simulink model "HA_sys7"  (R2017a)
settings: Solver=FixedStepDiscrete  StartTime=0.0  StopTime=stopTime  RelTol=1e-3
InitFcn:
  | HA_sys7_init
StopFcn:
  | %figure(1)
  | 
  | %subplot(2,1,1)
  | %plot(HA_left_data_out)
  | %title('Left Channel Output')
  | 
  | %subplot(2,1,2)
  | %plot(HA_right_data_out)
  | %title('Right Channel Output')
values from neighbouring files (symbols this model uses):
  Fs = 48000    [HA_sys7_init.m]
  Gain_B1_left = 1    [HA_sys7_init.m]
  Gain_B1_right = 1    [HA_sys7_init.m]
  Gain_B2_left = 1    [HA_sys7_init.m]
  Gain_B2_right = 1    [HA_sys7_init.m]
  Gain_B3_left = 1    [HA_sys7_init.m]
  Gain_B3_right = 1    [HA_sys7_init.m]
  Gain_B4_left = 1    [HA_sys7_init.m]
  Gain_B4_right = 1    [HA_sys7_init.m]
  Gain_B5_left = 1    [HA_sys7_init.m]
  Gain_B5_right = 1    [HA_sys7_init.m]
undefined symbols (not defined in the file or in its folder): FIRBandPass1, FIRBandPass2, FIRBandPass3, FIRBandPass4, FIRBandPass5, FIRDecimator1, FIRDecimator2, FIRDecimator3, FIRDecimator4, FIRDecimator5, FIRInterpolator1, FIRInterpolator2, FIRInterpolator3, FIRInterpolator4, FIRInterpolator5
libraries: dspmlti4 x20, dspsrcs4 x1
settings Model: DataTypeOverride=Off  Creator=The MathWorks, Inc.  LastModifiedBy=Ross_admin
settings DataIOCC: LimitDataPoints=on  SaveFormat=Array  SaveOutput=off  SaveTime=off
settings OptimizationCC: BlockReduction=off  ConditionallyExecuteInputs=off  DefaultParameterBehavior=Inlined  LifeSpan=inf
settings DebuggingCC: AlgebraicLoopMsg=error  SingleTaskRateTransMsg=error  AllowSymbolicDim=off  StrictBusMsg=ErrorOnBusTreatedAsVector  SFUnexpectedBacktrackingDiag=warning  SFNoUnconditionalDefaultTransitionDiag=warning  SFExecutionAtInitializationDiag=none
settings HardwareCC: ProdBitPerPointer=32  ProdBitPerSizeT=32  ProdBitPerPtrDiffT=32  ProdLargestAtomicFloat=None  ProdIntDivRoundTo=Undefined  ProdEndianess=Unspecified  ProdWordSize=32  ProdHWDeviceType=ASIC/FPGA->ASIC/FPGA  ProdEqTarget=off
settings ModelReferenceCC: PropagateSignalLabelsOutOfModel=off
settings GRTTargetCC: TargetLangStandard=C89/C90 (ANSI)  GeneratePreprocessorConditionals=Disable all
settings ConfigComp: CovMetricSettings=dw  CovHtmlReporting=on  CovSaveCumulativeToWorkspaceVar=on  CovSaveSingleToWorkspaceVar=on  CovShowResultsExplorer=off  CovExternalEMLEnable=off

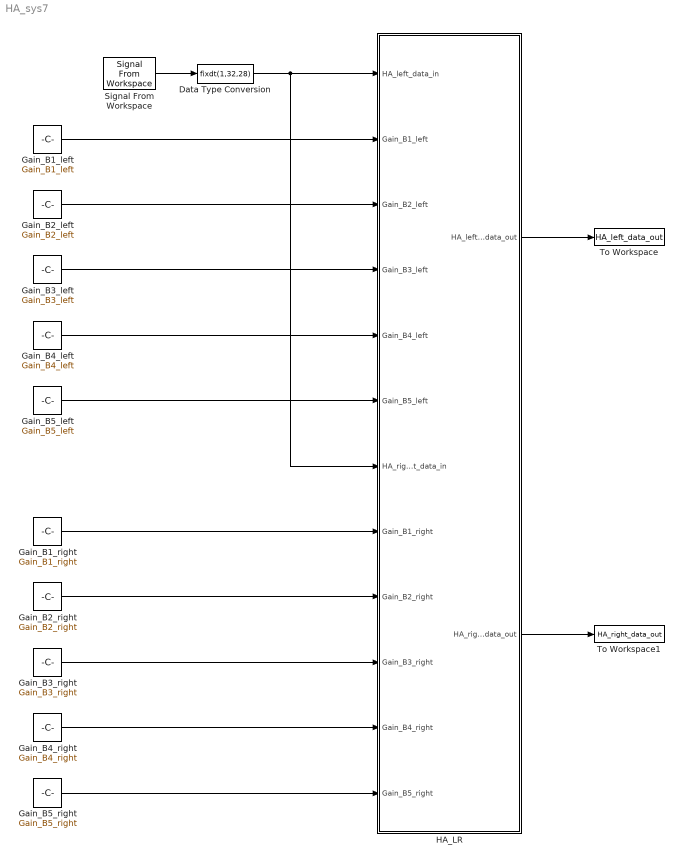
== system HA_sys7 ==
  Data Type Conversion : DataTypeConversion  OutDataTypeStr=fixdt(1,32,28)
  Gain_B1_left : Constant  Value=Gain_B1_left  OutDataTypeStr=fixdt(1,32,16)  SampleTime=-1  LockScale=on
  Gain_B1_right : Constant  Value=Gain_B1_right  OutDataTypeStr=fixdt(1,32,16)  SampleTime=-1  LockScale=on
  Gain_B2_left : Constant  Value=Gain_B2_left  OutDataTypeStr=fixdt(1,32,16)  SampleTime=-1  LockScale=on
  Gain_B2_right : Constant  Value=Gain_B2_right  OutDataTypeStr=fixdt(1,32,16)  SampleTime=-1  LockScale=on
  Gain_B3_left : Constant  Value=Gain_B3_left  OutDataTypeStr=fixdt(1,32,16)  SampleTime=-1  LockScale=on
  Gain_B3_right : Constant  Value=Gain_B3_right  OutDataTypeStr=fixdt(1,32,16)  SampleTime=-1  LockScale=on
  Gain_B4_left : Constant  Value=Gain_B4_left  OutDataTypeStr=fixdt(1,32,16)  SampleTime=-1  LockScale=on
  Gain_B4_right : Constant  Value=Gain_B4_right  OutDataTypeStr=fixdt(1,32,16)  SampleTime=-1  LockScale=on
  Gain_B5_left : Constant  Value=Gain_B5_left  OutDataTypeStr=fixdt(1,32,16)  SampleTime=-1  LockScale=on
  Gain_B5_right : Constant  Value=Gain_B5_right  OutDataTypeStr=fixdt(1,32,16)  SampleTime=-1  LockScale=on
  HA_LR : Subsystem
  Signal From Workspace : dspsrcs4/Signal From Workspace  X=signal_in  Ts=1/Fs  nsamps=1  OutputAfterFinalValue=Setting to zero  ignoreOrWarnInputAndFrameLengths=off  OutputFrames=off
  To Workspace : ToWorkspace  VariableName=HA_left_data_out  SampleTime=-1
      settings: Save2DSignal=2-D array (concatenate along first dimension)
  To Workspace1 : ToWorkspace  VariableName=HA_right_data_out  SampleTime=-1
      settings: Save2DSignal=2-D array (concatenate along first dimension)
  wires:
  Signal From Workspace/1 -> Data Type Conversion/1
  Data Type Conversion/1 -> HA_LR/7(HA_right_data_in), HA_LR/1(HA_left_data_in)
  Gain_B2_left/1 -> HA_LR/3(Gain_B2_left)
  Gain_B3_left/1 -> HA_LR/4(Gain_B3_left)
  Gain_B4_left/1 -> HA_LR/5(Gain_B4_left)
  Gain_B5_left/1 -> HA_LR/6(Gain_B5_left)
  HA_LR/1(HA_left_data_out) -> To Workspace/1
  HA_LR/2(HA_right_data_out) -> To Workspace1/1
  Gain_B1_left/1 -> HA_LR/2(Gain_B1_left)
  Gain_B1_right/1 -> HA_LR/8(Gain_B1_right)
  Gain_B2_right/1 -> HA_LR/9(Gain_B2_right)
  Gain_B4_right/1 -> HA_LR/11(Gain_B4_right)
  Gain_B5_right/1 -> HA_LR/12(Gain_B5_right)
  Gain_B3_right/1 -> HA_LR/10(Gain_B3_right)

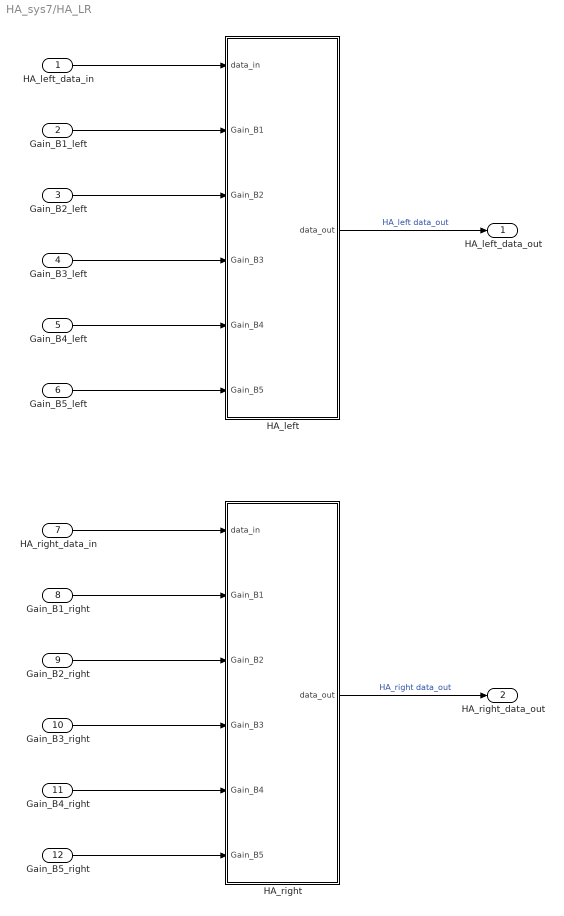
== system HA_sys7/HA_LR ==
  HA_left_data_in : Inport
  Gain_B1_left : Inport  Port=2
  Gain_B2_left : Inport  Port=3
  Gain_B3_left : Inport  Port=4
  Gain_B4_left : Inport  Port=5
  Gain_B5_left : Inport  Port=6
  HA_right_data_in : Inport  Port=7
  Gain_B1_right : Inport  Port=8
  Gain_B2_right : Inport  Port=9
  Gain_B3_right : Inport  Port=10
  Gain_B4_right : Inport  Port=11
  Gain_B5_right : Inport  Port=12
  HA_left : Subsystem
  HA_right : Subsystem
  HA_left_data_out : Outport
  HA_right_data_out : Outport  Port=2
  wires:
  Gain_B5_left/1 -> HA_left/6(Gain_B5)
  Gain_B4_left/1 -> HA_left/5(Gain_B4)
  Gain_B2_left/1 -> HA_left/3(Gain_B2)
  Gain_B3_left/1 -> HA_left/4(Gain_B3)
  Gain_B3_right/1 -> HA_right/4(Gain_B3)
  HA_right_data_in/1 -> HA_right/1(data_in)
  HA_right/1(data_out) -> HA_right_data_out/1  "HA_right data_out"
  Gain_B1_right/1 -> HA_right/2(Gain_B1)
  Gain_B2_right/1 -> HA_right/3(Gain_B2)
  Gain_B4_right/1 -> HA_right/5(Gain_B4)
  Gain_B5_right/1 -> HA_right/6(Gain_B5)
  HA_left_data_in/1 -> HA_left/1(data_in)
  HA_left/1(data_out) -> HA_left_data_out/1  "HA_left data_out"
  Gain_B1_left/1 -> HA_left/2(Gain_B1)

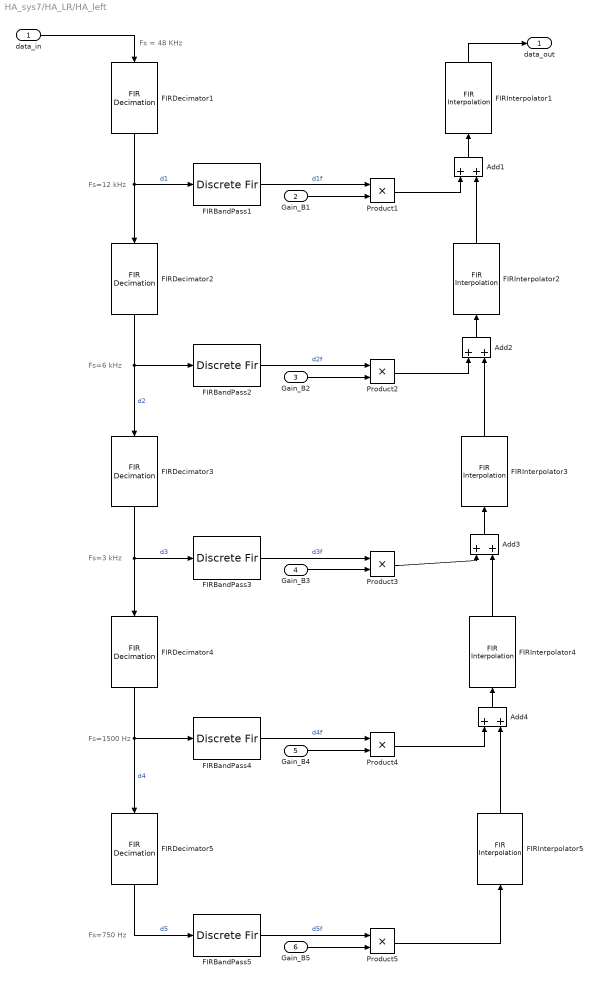
== system HA_sys7/HA_LR/HA_left ==
  note: Fs = 48 KHz
  note: Fs=12 kHz
  note: Fs=6 kHz
  note: Fs=3 kHz
  note: Fs=1500 Hz
  note: Fs=750 Hz
  data_in : Inport
  Gain_B1 : Inport  Port=2  OutDataTypeStr=fixdt(1,32,16)  LockScale=on
  Gain_B2 : Inport  Port=3  OutDataTypeStr=fixdt(1,32,16)  LockScale=on
  Gain_B3 : Inport  Port=4  OutDataTypeStr=fixdt(1,32,16)  LockScale=on
  Gain_B4 : Inport  Port=5  OutDataTypeStr=fixdt(1,32,16)  LockScale=on
  Gain_B5 : Inport  Port=6  OutDataTypeStr=fixdt(1,32,16)  LockScale=on
  Add{1..4} (4 alike) : Sum  SaturateOnIntegerOverflow=on
  FIRBandPass1 : DiscreteFir  Coefficients=FIRBandPass1.FIR_coefficients  AccumDataTypeStr=Inherit: Same as product output  SaturateOnIntegerOverflow=on
  FIRBandPass2 : DiscreteFir  Coefficients=FIRBandPass2.FIR_coefficients  AccumDataTypeStr=Inherit: Same as product output  OutDataTypeStr=FIRBandPass2.numeric_type  SaturateOnIntegerOverflow=on
  FIRBandPass3 : DiscreteFir  Coefficients=FIRBandPass3.FIR_coefficients  AccumDataTypeStr=Inherit: Same as product output  OutDataTypeStr=FIRBandPass2.numeric_type  SaturateOnIntegerOverflow=on
  FIRBandPass4 : DiscreteFir  Coefficients=FIRBandPass4.FIR_coefficients  AccumDataTypeStr=Inherit: Same as product output  OutDataTypeStr=FIRBandPass2.numeric_type  SaturateOnIntegerOverflow=on
  FIRBandPass5 : DiscreteFir  Coefficients=FIRBandPass5.FIR_coefficients  AccumDataTypeStr=Inherit: Same as product output  OutDataTypeStr=FIRBandPass2.numeric_type  SaturateOnIntegerOverflow=on
  FIRDecimator1 : dspmlti4/FIR Decimation  FilterSource=Dialog parameters  h=FIRDecimator1.FIR_coefficients  D=FIRDecimator1.decimation_factor  filtStruct=Direct form  FilterObject=FDECIM  framing=Allow multirate processing  inputOffset=0  outputBufInitCond=0  roundingMode=Floor  overflowMode=on  firstCoeffDataTypeStr=Inherit: Same word length as input  firstCoeffMin=[]  firstCoeffMax=[]  firstCoeffLastDataTypeStr=Inherit: Same word length as input  outputMode=Binary point scaling  outputWordLength=32  outputFracLength=28  outputDataTypeStr=fixdt(1,32,28)  outputMin=[]  outputMax=[]  outputLastDataTypeStr=fixdt(1,32,28)
  FIRDecimator2 : dspmlti4/FIR Decimation  FilterSource=Dialog parameters  h=FIRDecimator2.FIR_coefficients  D=FIRDecimator2.decimation_factor  filtStruct=Direct form  FilterObject=FDECIM  framing=Allow multirate processing  inputOffset=0  outputBufInitCond=0  roundingMode=Floor  overflowMode=on  firstCoeffDataTypeStr=Inherit: Same word length as input  firstCoeffMin=[]  firstCoeffMax=[]  firstCoeffLastDataTypeStr=Inherit: Same word length as input  outputMode=Binary point scaling  outputWordLength=32  outputFracLength=28  outputDataTypeStr=fixdt(1,32,28)  outputMin=[]  outputMax=[]  outputLastDataTypeStr=fixdt(1,32,28)
  FIRDecimator3 : dspmlti4/FIR Decimation  FilterSource=Dialog parameters  h=FIRDecimator3.FIR_coefficients  D=FIRDecimator3.decimation_factor  filtStruct=Direct form  FilterObject=FDECIM  framing=Allow multirate processing  inputOffset=0  outputBufInitCond=0  roundingMode=Floor  overflowMode=on  firstCoeffDataTypeStr=Inherit: Same word length as input  firstCoeffMin=[]  firstCoeffMax=[]  firstCoeffLastDataTypeStr=Inherit: Same word length as input  outputMode=Binary point scaling  outputWordLength=32  outputFracLength=28  outputDataTypeStr=fixdt(1,32,28)  outputMin=[]  outputMax=[]  outputLastDataTypeStr=fixdt(1,32,28)
  FIRDecimator4 : dspmlti4/FIR Decimation  FilterSource=Dialog parameters  h=FIRDecimator4.FIR_coefficients  D=FIRDecimator4.decimation_factor  filtStruct=Direct form  FilterObject=FDECIM  framing=Allow multirate processing  inputOffset=0  outputBufInitCond=0  roundingMode=Floor  overflowMode=on  firstCoeffDataTypeStr=Inherit: Same word length as input  firstCoeffMin=[]  firstCoeffMax=[]  firstCoeffLastDataTypeStr=Inherit: Same word length as input  outputMode=Binary point scaling  outputWordLength=32  outputFracLength=28  outputDataTypeStr=fixdt(1,32,28)  outputMin=[]  outputMax=[]  outputLastDataTypeStr=fixdt(1,32,28)
  FIRDecimator5 : dspmlti4/FIR Decimation  FilterSource=Dialog parameters  h=FIRDecimator5.FIR_coefficients  D=FIRDecimator5.decimation_factor  filtStruct=Direct form  FilterObject=FDECIM  framing=Allow multirate processing  inputOffset=0  outputBufInitCond=0  roundingMode=Floor  overflowMode=on  firstCoeffDataTypeStr=Inherit: Same word length as input  firstCoeffMin=[]  firstCoeffMax=[]  firstCoeffLastDataTypeStr=Inherit: Same word length as input  outputMode=Binary point scaling  outputWordLength=32  outputFracLength=28  outputDataTypeStr=fixdt(1,32,28)  outputMin=[]  outputMax=[]  outputLastDataTypeStr=fixdt(1,32,28)
  FIRInterpolator1 : dspmlti4/FIR Interpolation  FilterSource=Dialog parameters  h=FIRInterpolator1.FIR_coefficients  L=FIRInterpolator1.interpolation_factor  FilterObject=FINTERP  framing=Allow multirate processing  outputBufInitCond=0  roundingMode=Floor  overflowMode=on  firstCoeffDataTypeStr=Inherit: Same word length as input  firstCoeffMin=[]  firstCoeffMax=[]  firstCoeffLastDataTypeStr=Inherit: Same word length as input  outputMode=Binary point scaling  outputWordLength=32  outputFracLength=28  outputDataTypeStr=fixdt(1,32,28)  outputMin=[]  outputMax=[]  outputLastDataTypeStr=fixdt(1,32,28)
      settings: SourceProductName=DSP System Toolbox
  FIRInterpolator2 : dspmlti4/FIR Interpolation  FilterSource=Dialog parameters  h=FIRInterpolator2.FIR_coefficients  L=FIRInterpolator2.interpolation_factor  FilterObject=FINTERP  framing=Allow multirate processing  outputBufInitCond=0  roundingMode=Floor  overflowMode=on  firstCoeffDataTypeStr=Inherit: Same word length as input  firstCoeffMin=[]  firstCoeffMax=[]  firstCoeffLastDataTypeStr=Inherit: Same word length as input  outputMode=Binary point scaling  outputWordLength=32  outputFracLength=28  outputDataTypeStr=fixdt(1,32,28)  outputMin=[]  outputMax=[]  outputLastDataTypeStr=fixdt(1,32,28)
      settings: SourceProductName=DSP System Toolbox
  FIRInterpolator3 : dspmlti4/FIR Interpolation  FilterSource=Dialog parameters  h=FIRInterpolator3.FIR_coefficients  L=FIRInterpolator3.interpolation_factor  FilterObject=FINTERP  framing=Allow multirate processing  outputBufInitCond=0  roundingMode=Floor  overflowMode=on  firstCoeffDataTypeStr=Inherit: Same word length as input  firstCoeffMin=[]  firstCoeffMax=[]  firstCoeffLastDataTypeStr=Inherit: Same word length as input  outputMode=Binary point scaling  outputWordLength=32  outputFracLength=28  outputDataTypeStr=fixdt(1,32,28)  outputMin=[]  outputMax=[]  outputLastDataTypeStr=fixdt(1,32,28)
      settings: SourceProductName=DSP System Toolbox
  FIRInterpolator4 : dspmlti4/FIR Interpolation  FilterSource=Dialog parameters  h=FIRInterpolator4.FIR_coefficients  L=FIRInterpolator4.interpolation_factor  FilterObject=FINTERP  framing=Allow multirate processing  outputBufInitCond=0  roundingMode=Floor  overflowMode=on  firstCoeffDataTypeStr=Inherit: Same word length as input  firstCoeffMin=[]  firstCoeffMax=[]  firstCoeffLastDataTypeStr=Inherit: Same word length as input  outputMode=Binary point scaling  outputWordLength=32  outputFracLength=28  outputDataTypeStr=fixdt(1,32,28)  outputMin=[]  outputMax=[]  outputLastDataTypeStr=fixdt(1,32,28)
      settings: SourceProductName=DSP System Toolbox
  FIRInterpolator5 : dspmlti4/FIR Interpolation  FilterSource=Dialog parameters  h=FIRInterpolator5.FIR_coefficients  L=FIRInterpolator5.interpolation_factor  FilterObject=FINTERP  framing=Allow multirate processing  outputBufInitCond=0  roundingMode=Floor  overflowMode=on  firstCoeffDataTypeStr=Inherit: Same word length as input  firstCoeffMin=[]  firstCoeffMax=[]  firstCoeffLastDataTypeStr=Inherit: Same word length as input  outputMode=Binary point scaling  outputWordLength=32  outputFracLength=28  outputDataTypeStr=fixdt(1,32,28)  outputMin=[]  outputMax=[]  outputLastDataTypeStr=fixdt(1,32,28)
      settings: SourceProductName=DSP System Toolbox
  Product{1..5} (5 alike) : Product  OutDataTypeStr=fixdt(1,32,28)  SaturateOnIntegerOverflow=on
  data_out : Outport
  wires:
  data_in/1 -> FIRDecimator1/1
  FIRInterpolator1/1 -> data_out/1
  FIRDecimator1/1 -> FIRDecimator2/1, FIRBandPass1/1  "d1"
  FIRBandPass1/1 -> Product1/1  "d1f"
  Gain_B1/1 -> Product1/2
  Gain_B2/1 -> Product2/2
  FIRBandPass2/1 -> Product2/1  "d2f"
  FIRDecimator2/1 -> FIRDecimator3/1, FIRBandPass2/1  "d2"
  Add1/1 -> FIRInterpolator1/1
  Product1/1 -> Add1/1
  FIRInterpolator2/1 -> Add1/2
  FIRDecimator3/1 -> FIRDecimator4/1, FIRBandPass3/1  "d3"
  FIRBandPass3/1 -> Product3/1  "d3f"
  Gain_B3/1 -> Product3/2
  Add2/1 -> FIRInterpolator2/1
  Product2/1 -> Add2/1
  FIRInterpolator3/1 -> Add2/2
  FIRBandPass4/1 -> Product4/1  "d4f"
  Gain_B4/1 -> Product4/2
  FIRDecimator4/1 -> FIRDecimator5/1, FIRBandPass4/1  "d4"
  Add3/1 -> FIRInterpolator3/1
  Product3/1 -> Add3/1
  FIRInterpolator4/1 -> Add3/2
  FIRDecimator5/1 -> FIRBandPass5/1  "d5"
  Gain_B5/1 -> Product5/2
  FIRBandPass5/1 -> Product5/1  "d5f"
  Product5/1 -> FIRInterpolator5/1
  Add4/1 -> FIRInterpolator4/1
  Product4/1 -> Add4/1
  FIRInterpolator5/1 -> Add4/2

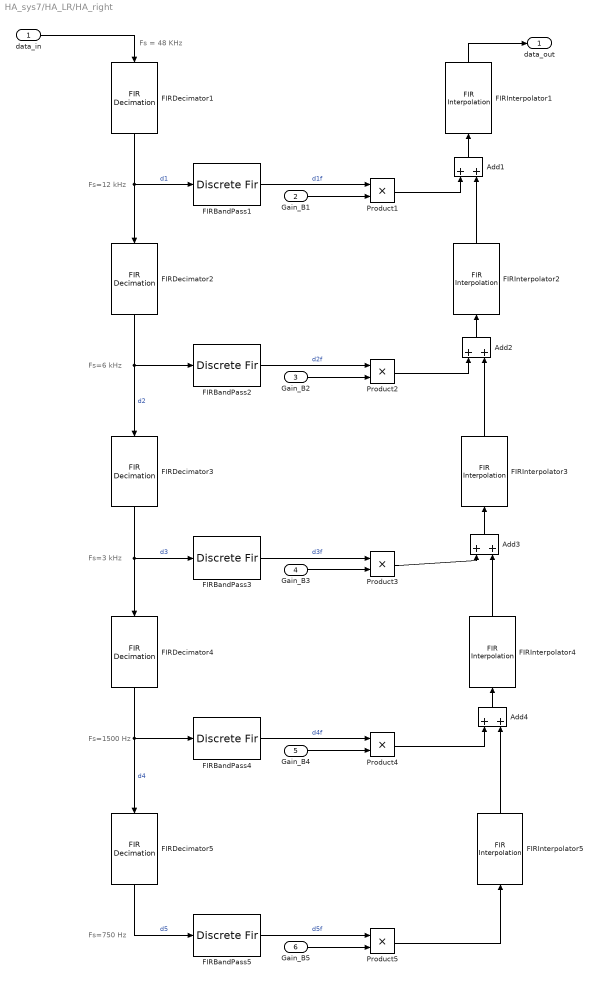
== system HA_sys7/HA_LR/HA_right ==
  note: Fs = 48 KHz
  note: Fs=12 kHz
  note: Fs=6 kHz
  note: Fs=3 kHz
  note: Fs=1500 Hz
  note: Fs=750 Hz
  data_in : Inport
  Gain_B1 : Inport  Port=2  OutDataTypeStr=fixdt(1,32,16)  LockScale=on
  Gain_B2 : Inport  Port=3  OutDataTypeStr=fixdt(1,32,16)  LockScale=on
  Gain_B3 : Inport  Port=4  OutDataTypeStr=fixdt(1,32,16)  LockScale=on
  Gain_B4 : Inport  Port=5  OutDataTypeStr=fixdt(1,32,16)  LockScale=on
  Gain_B5 : Inport  Port=6  OutDataTypeStr=fixdt(1,32,16)  LockScale=on
  Add{1..4} (4 alike) : Sum  SaturateOnIntegerOverflow=on
  FIRBandPass1 : DiscreteFir  Coefficients=FIRBandPass1.FIR_coefficients  AccumDataTypeStr=Inherit: Same as product output  SaturateOnIntegerOverflow=on
  FIRBandPass2 : DiscreteFir  Coefficients=FIRBandPass2.FIR_coefficients  AccumDataTypeStr=Inherit: Same as product output  OutDataTypeStr=FIRBandPass2.numeric_type  SaturateOnIntegerOverflow=on
  FIRBandPass3 : DiscreteFir  Coefficients=FIRBandPass3.FIR_coefficients  AccumDataTypeStr=Inherit: Same as product output  OutDataTypeStr=FIRBandPass2.numeric_type  SaturateOnIntegerOverflow=on
  FIRBandPass4 : DiscreteFir  Coefficients=FIRBandPass4.FIR_coefficients  AccumDataTypeStr=Inherit: Same as product output  OutDataTypeStr=FIRBandPass2.numeric_type  SaturateOnIntegerOverflow=on
  FIRBandPass5 : DiscreteFir  Coefficients=FIRBandPass5.FIR_coefficients  AccumDataTypeStr=Inherit: Same as product output  OutDataTypeStr=FIRBandPass2.numeric_type  SaturateOnIntegerOverflow=on
  FIRDecimator1 : dspmlti4/FIR Decimation  FilterSource=Dialog parameters  h=FIRDecimator1.FIR_coefficients  D=FIRDecimator1.decimation_factor  filtStruct=Direct form  FilterObject=FDECIM  framing=Allow multirate processing  inputOffset=0  outputBufInitCond=0  roundingMode=Floor  overflowMode=on  firstCoeffDataTypeStr=Inherit: Same word length as input  firstCoeffMin=[]  firstCoeffMax=[]  firstCoeffLastDataTypeStr=Inherit: Same word length as input  outputMode=Binary point scaling  outputWordLength=32  outputFracLength=28  outputDataTypeStr=fixdt(1,32,28)  outputMin=[]  outputMax=[]  outputLastDataTypeStr=fixdt(1,32,28)
  FIRDecimator2 : dspmlti4/FIR Decimation  FilterSource=Dialog parameters  h=FIRDecimator2.FIR_coefficients  D=FIRDecimator2.decimation_factor  filtStruct=Direct form  FilterObject=FDECIM  framing=Allow multirate processing  inputOffset=0  outputBufInitCond=0  roundingMode=Floor  overflowMode=on  firstCoeffDataTypeStr=Inherit: Same word length as input  firstCoeffMin=[]  firstCoeffMax=[]  firstCoeffLastDataTypeStr=Inherit: Same word length as input  outputMode=Binary point scaling  outputWordLength=32  outputFracLength=28  outputDataTypeStr=fixdt(1,32,28)  outputMin=[]  outputMax=[]  outputLastDataTypeStr=fixdt(1,32,28)
  FIRDecimator3 : dspmlti4/FIR Decimation  FilterSource=Dialog parameters  h=FIRDecimator3.FIR_coefficients  D=FIRDecimator3.decimation_factor  filtStruct=Direct form  FilterObject=FDECIM  framing=Allow multirate processing  inputOffset=0  outputBufInitCond=0  roundingMode=Floor  overflowMode=on  firstCoeffDataTypeStr=Inherit: Same word length as input  firstCoeffMin=[]  firstCoeffMax=[]  firstCoeffLastDataTypeStr=Inherit: Same word length as input  outputMode=Binary point scaling  outputWordLength=32  outputFracLength=28  outputDataTypeStr=fixdt(1,32,28)  outputMin=[]  outputMax=[]  outputLastDataTypeStr=fixdt(1,32,28)
  FIRDecimator4 : dspmlti4/FIR Decimation  FilterSource=Dialog parameters  h=FIRDecimator4.FIR_coefficients  D=FIRDecimator4.decimation_factor  filtStruct=Direct form  FilterObject=FDECIM  framing=Allow multirate processing  inputOffset=0  outputBufInitCond=0  roundingMode=Floor  overflowMode=on  firstCoeffDataTypeStr=Inherit: Same word length as input  firstCoeffMin=[]  firstCoeffMax=[]  firstCoeffLastDataTypeStr=Inherit: Same word length as input  outputMode=Binary point scaling  outputWordLength=32  outputFracLength=28  outputDataTypeStr=fixdt(1,32,28)  outputMin=[]  outputMax=[]  outputLastDataTypeStr=fixdt(1,32,28)
  FIRDecimator5 : dspmlti4/FIR Decimation  FilterSource=Dialog parameters  h=FIRDecimator5.FIR_coefficients  D=FIRDecimator5.decimation_factor  filtStruct=Direct form  FilterObject=FDECIM  framing=Allow multirate processing  inputOffset=0  outputBufInitCond=0  roundingMode=Floor  overflowMode=on  firstCoeffDataTypeStr=Inherit: Same word length as input  firstCoeffMin=[]  firstCoeffMax=[]  firstCoeffLastDataTypeStr=Inherit: Same word length as input  outputMode=Binary point scaling  outputWordLength=32  outputFracLength=28  outputDataTypeStr=fixdt(1,32,28)  outputMin=[]  outputMax=[]  outputLastDataTypeStr=fixdt(1,32,28)
  FIRInterpolator1 : dspmlti4/FIR Interpolation  FilterSource=Dialog parameters  h=FIRInterpolator1.FIR_coefficients  L=FIRInterpolator1.interpolation_factor  FilterObject=FINTERP  framing=Allow multirate processing  outputBufInitCond=0  roundingMode=Floor  overflowMode=on  firstCoeffDataTypeStr=Inherit: Same word length as input  firstCoeffMin=[]  firstCoeffMax=[]  firstCoeffLastDataTypeStr=Inherit: Same word length as input  outputMode=Binary point scaling  outputWordLength=32  outputFracLength=28  outputDataTypeStr=fixdt(1,32,28)  outputMin=[]  outputMax=[]  outputLastDataTypeStr=fixdt(1,32,28)
      settings: SourceProductName=DSP System Toolbox
  FIRInterpolator2 : dspmlti4/FIR Interpolation  FilterSource=Dialog parameters  h=FIRInterpolator2.FIR_coefficients  L=FIRInterpolator2.interpolation_factor  FilterObject=FINTERP  framing=Allow multirate processing  outputBufInitCond=0  roundingMode=Floor  overflowMode=on  firstCoeffDataTypeStr=Inherit: Same word length as input  firstCoeffMin=[]  firstCoeffMax=[]  firstCoeffLastDataTypeStr=Inherit: Same word length as input  outputMode=Binary point scaling  outputWordLength=32  outputFracLength=28  outputDataTypeStr=fixdt(1,32,28)  outputMin=[]  outputMax=[]  outputLastDataTypeStr=fixdt(1,32,28)
      settings: SourceProductName=DSP System Toolbox
  FIRInterpolator3 : dspmlti4/FIR Interpolation  FilterSource=Dialog parameters  h=FIRInterpolator3.FIR_coefficients  L=FIRInterpolator3.interpolation_factor  FilterObject=FINTERP  framing=Allow multirate processing  outputBufInitCond=0  roundingMode=Floor  overflowMode=on  firstCoeffDataTypeStr=Inherit: Same word length as input  firstCoeffMin=[]  firstCoeffMax=[]  firstCoeffLastDataTypeStr=Inherit: Same word length as input  outputMode=Binary point scaling  outputWordLength=32  outputFracLength=28  outputDataTypeStr=fixdt(1,32,28)  outputMin=[]  outputMax=[]  outputLastDataTypeStr=fixdt(1,32,28)
      settings: SourceProductName=DSP System Toolbox
  FIRInterpolator4 : dspmlti4/FIR Interpolation  FilterSource=Dialog parameters  h=FIRInterpolator4.FIR_coefficients  L=FIRInterpolator4.interpolation_factor  FilterObject=FINTERP  framing=Allow multirate processing  outputBufInitCond=0  roundingMode=Floor  overflowMode=on  firstCoeffDataTypeStr=Inherit: Same word length as input  firstCoeffMin=[]  firstCoeffMax=[]  firstCoeffLastDataTypeStr=Inherit: Same word length as input  outputMode=Binary point scaling  outputWordLength=32  outputFracLength=28  outputDataTypeStr=fixdt(1,32,28)  outputMin=[]  outputMax=[]  outputLastDataTypeStr=fixdt(1,32,28)
      settings: SourceProductName=DSP System Toolbox
  FIRInterpolator5 : dspmlti4/FIR Interpolation  FilterSource=Dialog parameters  h=FIRInterpolator5.FIR_coefficients  L=FIRInterpolator5.interpolation_factor  FilterObject=FINTERP  framing=Allow multirate processing  outputBufInitCond=0  roundingMode=Floor  overflowMode=on  firstCoeffDataTypeStr=Inherit: Same word length as input  firstCoeffMin=[]  firstCoeffMax=[]  firstCoeffLastDataTypeStr=Inherit: Same word length as input  outputMode=Binary point scaling  outputWordLength=32  outputFracLength=28  outputDataTypeStr=fixdt(1,32,28)  outputMin=[]  outputMax=[]  outputLastDataTypeStr=fixdt(1,32,28)
      settings: SourceProductName=DSP System Toolbox
  Product{1..5} (5 alike) : Product  OutDataTypeStr=fixdt(1,32,28)  SaturateOnIntegerOverflow=on
  data_out : Outport
  wires:
  data_in/1 -> FIRDecimator1/1
  FIRInterpolator1/1 -> data_out/1
  FIRDecimator1/1 -> FIRDecimator2/1, FIRBandPass1/1  "d1"
  FIRBandPass1/1 -> Product1/1  "d1f"
  Gain_B1/1 -> Product1/2
  Gain_B2/1 -> Product2/2
  FIRBandPass2/1 -> Product2/1  "d2f"
  FIRDecimator2/1 -> FIRDecimator3/1, FIRBandPass2/1  "d2"
  Add1/1 -> FIRInterpolator1/1
  Product1/1 -> Add1/1
  FIRInterpolator2/1 -> Add1/2
  FIRDecimator3/1 -> FIRDecimator4/1, FIRBandPass3/1  "d3"
  FIRBandPass3/1 -> Product3/1  "d3f"
  Gain_B3/1 -> Product3/2
  Add2/1 -> FIRInterpolator2/1
  Product2/1 -> Add2/1
  FIRInterpolator3/1 -> Add2/2
  FIRBandPass4/1 -> Product4/1  "d4f"
  Gain_B4/1 -> Product4/2
  FIRDecimator4/1 -> FIRDecimator5/1, FIRBandPass4/1  "d4"
  Add3/1 -> FIRInterpolator3/1
  Product3/1 -> Add3/1
  FIRInterpolator4/1 -> Add3/2
  FIRDecimator5/1 -> FIRBandPass5/1  "d5"
  Gain_B5/1 -> Product5/2
  FIRBandPass5/1 -> Product5/1  "d5f"
  Product5/1 -> FIRInterpolator5/1
  Add4/1 -> FIRInterpolator4/1
  Product4/1 -> Add4/1
  FIRInterpolator5/1 -> Add4/2
